simulink model "OCTModelLateralFlight"  (R2018b)
settings: Solver=FixedStepAuto  StartTime=0.0  StopTime=duration_s  FixedStep=0.1  MaxStep=0.1  RelTol=1e-3  AbsTol=1e-3
libraries: environment_cl x1, lateralFlightController x1, plant_cl x1
settings Model: ExtModeTrigDuration=100  Creator=mcobb  LastModifiedBy=jldanie5
settings DataIOCC: SaveOutput=off  StateSaveName=tmp_raccel_xout
settings OptimizationCC: EfficientMapNaN2IntZero=off
settings DebuggingCC: SignalRangeChecking=error
settings HardwareCC: TargetBitPerPointer=64  TargetBitPerSizeT=64  TargetBitPerPtrDiffT=64  TargetLongLongMode=on  TargetIntDivRoundTo=Zero  TargetEndianess=LittleEndian  TargetWordSize=64  TargetHWDeviceType=MATLAB Host  ProdEqTarget=off
settings RTWCC: SystemTargetFile=raccel.tlc  TemplateMakefile=raccel_default_tmf  RTWVerbose=off  RTWUseSimCustomCode=on
settings CodeAppCC: GenerateComments=off  MaxIdLength=128  MangleLength=10
settings RaccelTargetCC: GeneratePreprocessorConditionals=Use local settings  MultiInstanceERTCode=off  PreserveStateflowLocalDataDimensions=off  ENABLE_SLEXEC_SSBRIDGE=1  RTWCAPIParams=on

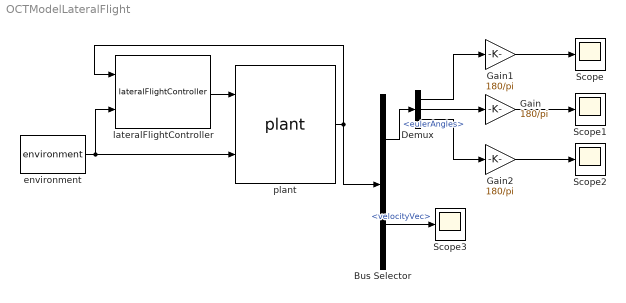
== system OCTModelLateralFlight ==
  Bus Selector : BusSelector  OutputSignals=eulerAngles,velocityVec
  Demux : Demux  Outputs=3
  Gain : Gain  Gain=180/pi
  Gain1 : Gain  Gain=180/pi
  Gain2 : Gain  Gain=180/pi
  Scope{,1..3} (4 alike) : Scope
  environment : environment_cl/environment  SystemSampleTime=-1
  lateralFlightController : lateralFlightController/lateralFlightController  SystemSampleTime=-1
  plant : plant_cl/plant  SystemSampleTime=-1  VariantControl=VSS_plant_modularPlant
      link override vehicle/modVehicle000: rho=env.water.density.Value  grav=env.gravAccel.Value
  wires:
  lateralFlightController/1 -> plant/1
  plant/1 -> lateralFlightController/1, Bus Selector/1
  environment/1 -> lateralFlightController/2, plant/2
  Bus Selector/1 -> Demux/1  "<eulerAngles>"
  Demux/2 -> Gain/1
  Gain/1 -> Scope1/1
  Bus Selector/2 -> Scope3/1  "<velocityVec>"
  Gain2/1 -> Scope2/1
  Gain1/1 -> Scope/1
  Demux/1 -> Gain1/1
  Demux/3 -> Gain2/1
